simulink model "DroneModel"  (R2023a)
settings: Solver=VariableStepAuto  StartTime=0.0  StopTime=10  RelTol=1e-3
values from neighbouring files (symbols this model uses):
  b = 0.11    [quadraptorModel.m]
  I = diag([Ixx, Iyy, Izz])    [quadraptorModel.m]
  k = 2.165856918e-8    (= 2.165856918e-08)    [quadraptorModel.m]
  L = 0.0475    [quadraptorModel.m]
  m = drone_mass + optitrack_frame_mass    (= 0.067)    [quadraptorModel.m]
  mg = [0; 0; m * g]    [quadraptorModel.m]
  motor_max_rpm = 24000    [quadraptorModel.m]
libraries: slpidlib x2, matrix_library x1
settings Model: Creator=enriq  LastModifiedBy=enriq

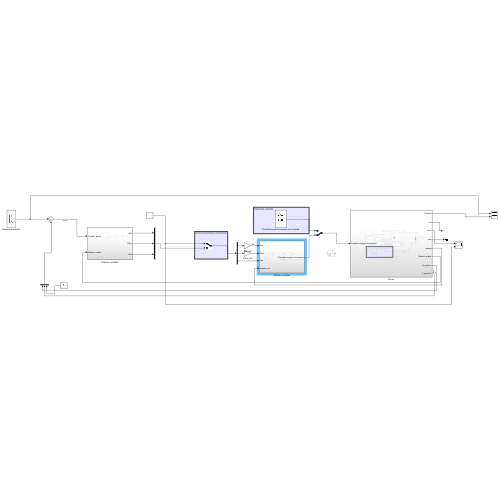
[thumbnail: Simulink's stored preview of the top-level diagram]
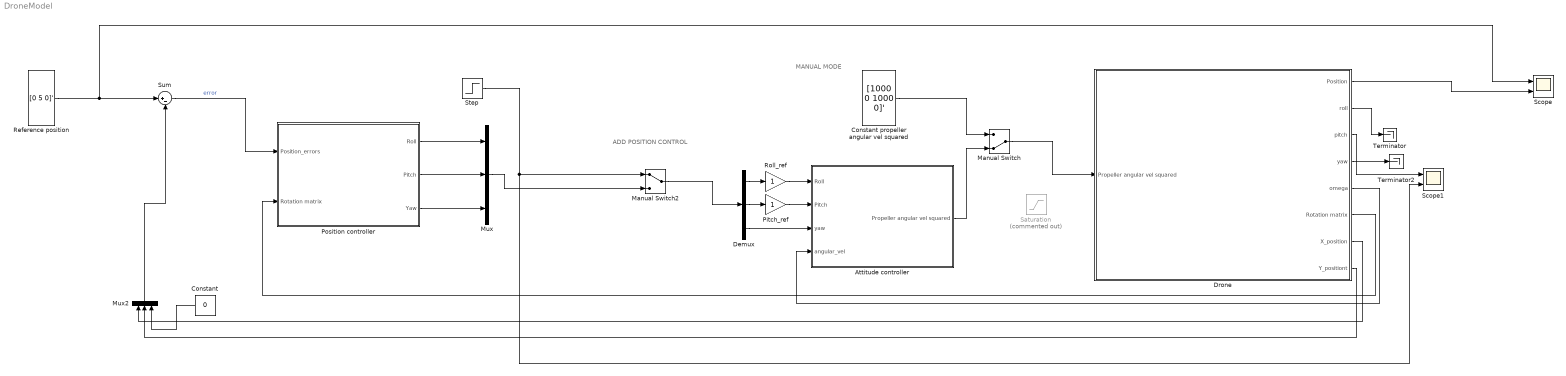
== system DroneModel ==
  note: ADD POSITION CONTROL
  note: MANUAL MODE
  Attitude controller : Subsystem
  Constant : Constant  Value=0
  Constant propeller angular vel squared : Constant  Value=[1000 0 1000 0]'  VectorParams1D=off
  Demux : Demux  Outputs=3
  Drone : Subsystem
  Manual Switch : ManualSwitch  CurrentSetting=0
  Manual Switch2 : ManualSwitch
  Mux : Mux  Inputs=3
  Mux2 : Mux  Inputs=3
  Pitch_ref : Gain
  Position controller : Subsystem
  Reference position : Constant  Value=[0 5 0]'  VectorParams1D=off
  Roll_ref : Gain
  Saturation : Saturate  Commented=on  UpperLimit=motor_max_rpm * (60/(2*pi))
  Scope : Scope  NumInputPorts=2
  Scope1 : Scope  NumInputPorts=2
  Step : Step  Before=[0; 0; 0]  After=[0; 1; 0]  SampleTime=0  VectorParams1D=off
  Sum : Sum  Inputs=|+-
  Terminator : Terminator
  Terminator2 : Terminator
  wires:
  Drone/1(Position) -> Scope/2
  Drone/2(roll) -> Terminator/1
  Drone/4(yaw) -> Terminator2/1
  Reference position/1 -> Scope/1, Sum/1
  Sum/1 -> Position controller/1(Position_errors)  "error"
  Constant propeller angular vel squared/1 -> Manual Switch/1
  Attitude controller/1(Propeller angular vel squared) -> Manual Switch/2
  Drone/5(omega) -> Attitude controller/4(angular_vel)
  Demux/1 -> Roll_ref/1
  Demux/2 -> Pitch_ref/1
  Demux/3 -> Attitude controller/3(yaw)
  Step/1 -> Manual Switch2/1, Scope1/2
  Drone/3(pitch) -> Scope1/1
  Drone/6(Rotation matrix) -> Position controller/2(Rotation matrix)
  Manual Switch2/1 -> Demux/1
  Position controller/1(Roll) -> Mux/1
  Position controller/2(Pitch) -> Mux/2
  Position controller/3(Yaw) -> Mux/3
  Mux/1 -> Manual Switch2/2
  Drone/8(Y_positiont) -> Mux2/2
  Drone/7(X_position) -> Mux2/1
  Constant/1 -> Mux2/3
  Mux2/1 -> Sum/2
  Pitch_ref/1 -> Attitude controller/2(Pitch)
  Roll_ref/1 -> Attitude controller/1(Roll)
  Manual Switch/1 -> Drone/1(Propeller angular vel squared)

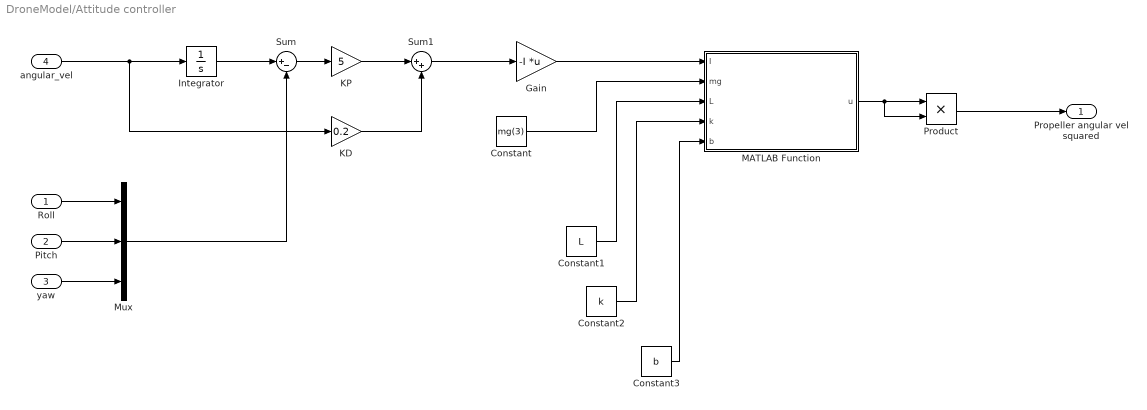
== system DroneModel/Attitude controller ==
  Roll : Inport
  Pitch : Inport  Port=2
  yaw : Inport  Port=3
  angular_vel : Inport  Port=4
  Constant : Constant  Value=mg(3)
  Constant1 : Constant  Value=L
  Constant2 : Constant  Value=k
  Constant3 : Constant  Value=b
  Gain : Gain  Gain=-I  Multiplication=Matrix(K*u)
  Integrator : Integrator
  KD : Gain  Gain=0.2
  KP : Gain  Gain=5
  MATLAB Function : MATLAB Function  TreatAsAtomicUnit=on
  Mux : Mux  Inputs=3
  Product : Product
  Sum : Sum  Inputs=|+-
  Sum1 : Sum  Inputs=|++
  Propeller angular vel squared : Outport
  wires:
  angular_vel/1 -> KD/1, Integrator/1
  Roll/1 -> Mux/1
  Pitch/1 -> Mux/2
  yaw/1 -> Mux/3
  Integrator/1 -> Sum/1
  Mux/1 -> Sum/2
  Sum/1 -> KP/1
  KP/1 -> Sum1/1
  KD/1 -> Sum1/2
  Sum1/1 -> Gain/1
  Gain/1 -> MATLAB Function/1(I)
  Constant1/1 -> MATLAB Function/3(L)
  Constant2/1 -> MATLAB Function/4(k)
  Constant3/1 -> MATLAB Function/5(b)
  MATLAB Function/1(u) -> Product/2, Product/1
  Product/1 -> Propeller angular vel squared/1
  Constant/1 -> MATLAB Function/2(mg)

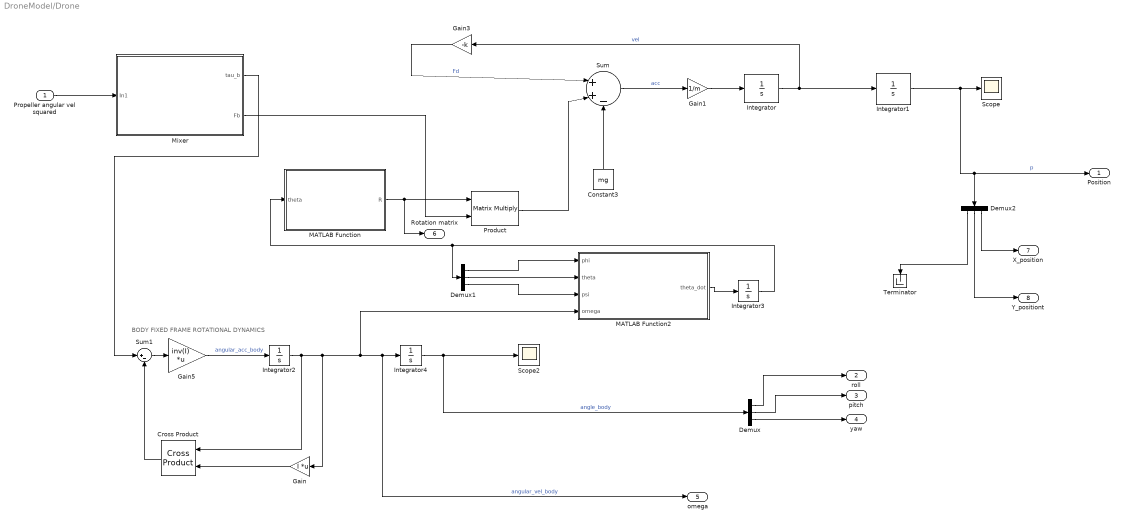
== system DroneModel/Drone ==
  note: BODY FIXED FRAME ROTATIONAL DYNAMICS
  Propeller angular vel squared : Inport
  Constant3 : Constant  Value=mg
  Cross Product : matrix_library/Cross Product
  Demux : Demux  Outputs=3
  Demux1 : Demux  Outputs=3
  Demux2 : Demux  Outputs=3
  Gain : Gain  Gain=I  Multiplication=Matrix(K*u)
  Gain1 : Gain  Gain=1/m
  Gain3 : Gain  Gain=-k
  Gain5 : Gain  Gain=inv(I)  Multiplication=Matrix(K*u)
  Integrator{,1..4} (5 alike) : Integrator
  MATLAB Function : MATLAB Function  TreatAsAtomicUnit=on
  MATLAB Function2 : MATLAB Function  TreatAsAtomicUnit=on
  Mixer : Subsystem
  Product : Product  Multiplication=Matrix(*)
  Scope : Scope
  Scope2 : Scope
  Sum : Sum  Inputs=|++-
  Sum1 : Sum  Inputs=|+-
  Terminator : Terminator
  Position : Outport
  roll : Outport  Port=2
  pitch : Outport  Port=3
  yaw : Outport  Port=4
  omega : Outport  Port=5
  Rotation matrix : Outport  Port=6
  X_position : Outport  Port=7
  Y_positiont : Outport  Port=8
  wires:
  Integrator2/1 -> MATLAB Function2/4(omega), omega/1, Integrator4/1, Gain/1, Cross Product/1  "angular_vel_body"
  Sum1/1 -> Gain5/1
  Mixer/1(tau_b) -> Sum1/1
  Integrator1/1 -> Demux2/1, Position/1, Scope/1  "p"
  Integrator/1 -> Gain3/1, Integrator1/1  "vel"
  Gain/1 -> Cross Product/2
  Integrator3/1 -> Demux1/1, MATLAB Function/1(theta)
  Sum/1 -> Gain1/1  "acc"
  Gain1/1 -> Integrator/1
  Constant3/1 -> Sum/3
  Demux/1 -> roll/1
  Demux/2 -> pitch/1
  Demux/3 -> yaw/1
  Propeller angular vel squared/1 -> Mixer/1(In1)
  MATLAB Function/1(R) -> Rotation matrix/1, Product/1
  Mixer/2(Fb) -> Product/2
  Product/1 -> Sum/2
  Gain3/1 -> Sum/1  "Fd"
  Gain5/1 -> Integrator2/1  "angular_acc_body"
  Cross Product/1 -> Sum1/2
  Integrator4/1 -> Demux/1, Scope2/1  "angle_body"
  MATLAB Function2/1(theta_dot) -> Integrator3/1
  Demux1/1 -> MATLAB Function2/1(phi)
  Demux1/2 -> MATLAB Function2/2(theta)
  Demux1/3 -> MATLAB Function2/3(psi)
  Demux2/3 -> X_position/1
  Demux2/2 -> Y_positiont/1
  Demux2/1 -> Terminator/1

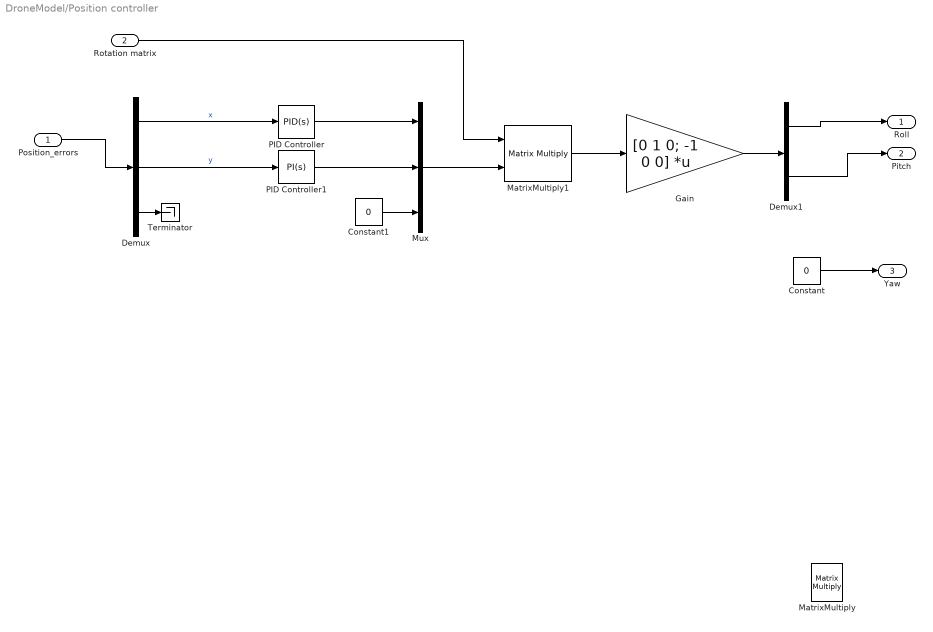
== system DroneModel/Position controller ==
  Position_errors : Inport
  Rotation matrix : Inport  Port=2
  Constant : Constant  Value=0
  Constant1 : Constant  Value=0
  Demux : Demux  Outputs=3
  Demux1 : Demux  Outputs=2
  Gain : Gain  Gain=[0 1 0; -1 0 0]  Multiplication=Matrix(K*u)
  MatrixMultiply : Product  Multiplication=Matrix(*)
  MatrixMultiply1 : Product  Multiplication=Matrix(*)
  Mux : Mux  Inputs=3
  PID Controller : slpidlib/PID Controller  Controller=PID  Form=Parallel  TimeDomain=Continuous-time  UseExternalTs=off  SampleTime=-1  IntegratorMethod=Forward Euler  FilterMethod=Forward Euler  ControllerParametersSource=internal  P=1  I=1  UseKiTs=off  D=0  N=100  UseFilter=on  TunerSelectOption=Transfer Function Based (PID Tuner App)  InitialConditionSource=internal  InitialConditionForIntegrator=0  InitialConditionForFilter=0  DifferentiatorICPrevScaledInput=0  ExternalReset=none  TrackingMode=off  Kt=1  LimitOutput=off  SatLimitsSource=internal  UpperSaturationLimit=inf  LowerSaturationLimit=-inf  LinearizeAsGain=on  AntiWindupMode=none  Kb=1  LimitIntegrator=off  UpperIntegratorSaturationLimit=inf  LowerIntegratorSaturationLimit=-inf  POutMin=[]  POutMax=[]  IOutMin=[]  IOutMax=[]  DOutMin=[]  DOutMax=[]  NOutMin=[]  NOutMax=[]  SumOutMin=[]  SumOutMax=[]  SaturationOutMin=[]  SaturationOutMax=[]  PParamMin=[]  PParamMax=[]  IParamMin=[]  IParamMax=[]  DParamMin=[]  DParamMax=[]  NParamMin=[]  NParamMax=[]  KbParamMin=[]  KbParamMax=[]  KtParamMin=[]  KtParamMax=[]  KbOutMin=[]  KbOutMax=[]  KtOutMin=[]  KtOutMax=[]  IntegratorOutMin=[]  IntegratorOutMax=[]  FilterOutMin=[]  FilterOutMax=[]  SumI1OutMin=[]  SumI1OutMax=[]  SumI2OutMin=[]  SumI2OutMax=[]  SumI3OutMin=[]  SumI3OutMax=[]  SumI4OutMin=[]  SumI4OutMax=[]  SumDOutMin=[]  SumDOutMax=[]  DifferentiatorOutMin=[]  DifferentiatorOutMax=[]  FilterDiffOutCoefMin=[]  FilterDiffOutCoefMax=[]  ReciprocalOutMin=[]  ReciprocalOutMax=[]  SumDenOutMin=[]  SumDenOutMax=[]  SumNumOutMin=[]  SumNumOutMax=[]  DivideOutMin=[]  DivideOutMax=[]  UdiffTsProdOutMin=[]  UdiffTsProdOutMax=[]  NTsProdOutMin=[]  NTsProdOutMax=[]  UintegralTsProdOutMin=[]  UintegralTsProdOutMax=[]  UngainTsProdOutMin=[]  UngainTsProdOutMax=[]  ClampingZeroOutDataTypeStr=Inherit: Inherit via back propagation  ClampingZeroOutMin=[]  ClampingZeroOutMax=[]  FilterDenConstantOutDataTypeStr=Inherit: Inherit via back propagation  FilterDenConstantOutMin=[]  FilterDenConstantOutMax=[]  PCopyOutDataTypeStr=Inherit: Inherit via back propagation  PCopyOutMin=[]  PCopyOutMax=[]  NCopyOutDataTypeStr=Inherit: Inherit via back propagation  NCopyOutMin=[]  NCopyOutMax=[]  IntegratorContinuousStateAttributes=''  IntegratorStateMustResolveToSignalObject=off  IntegratorRTWStateStorageClass=Auto  FilterContinuousStateAttributes=''  FilterStateMustResolveToSignalObject=off  FilterRTWStateStorageClass=Auto  ParallelPVariant=InternalParameters  IdealPVariant=Disabled  IVariant=InternalParameters  DVariant=InternalParameters  IntegratorVariant=Continuous  SatVariant=Disabled  AWVariant=Passthrough  PCopyVariant=Disabled  TRVariant=Disabled  FdbkBlocksVariant=Forward  IdealPFdbkVariant=Disabled  SatFdbkVariant=Disabled  DerivativeFilterVariant=ContFilter  NVariant=InternalParameters  NCopyVariant=Disabled  FilterICVariant=InternalICsFilter  IntegratorICVariant=InternalICs  ExternalResetVariant=Disabled  TRSumVariant=Passthrough  SumFdbkVariant=Disabled  SumVariant=Sum_PID  TsampFilterVariant=InternalTs  TsampNgainVariant=Passthrough  TsampIntegralVariant=Disabled_SignalSpec  ExternalSaturationOutDataTypeStr=Inherit: Same as second input
  PID Controller1 : slpidlib/PID Controller  Controller=PI  Form=Parallel  TimeDomain=Continuous-time  UseExternalTs=off  SampleTime=-1  IntegratorMethod=Forward Euler  FilterMethod=Forward Euler  ControllerParametersSource=internal  P=4.65  I=1  UseKiTs=off  D=0  N=100  UseFilter=on  TunerSelectOption=Transfer Function Based (PID Tuner App)  InitialConditionSource=internal  InitialConditionForIntegrator=0  InitialConditionForFilter=0  DifferentiatorICPrevScaledInput=0  ExternalReset=none  TrackingMode=off  Kt=1  LimitOutput=off  SatLimitsSource=internal  UpperSaturationLimit=inf  LowerSaturationLimit=-inf  LinearizeAsGain=on  AntiWindupMode=none  Kb=1  LimitIntegrator=off  UpperIntegratorSaturationLimit=inf  LowerIntegratorSaturationLimit=-inf  POutMin=[]  POutMax=[]  IOutMin=[]  IOutMax=[]  DOutMin=[]  DOutMax=[]  NOutMin=[]  NOutMax=[]  SumOutMin=[]  SumOutMax=[]  SaturationOutMin=[]  SaturationOutMax=[]  PParamMin=[]  PParamMax=[]  IParamMin=[]  IParamMax=[]  DParamMin=[]  DParamMax=[]  NParamMin=[]  NParamMax=[]  KbParamMin=[]  KbParamMax=[]  KtParamMin=[]  KtParamMax=[]  KbOutMin=[]  KbOutMax=[]  KtOutMin=[]  KtOutMax=[]  IntegratorOutMin=[]  IntegratorOutMax=[]  FilterOutMin=[]  FilterOutMax=[]  SumI1OutMin=[]  SumI1OutMax=[]  SumI2OutMin=[]  SumI2OutMax=[]  SumI3OutMin=[]  SumI3OutMax=[]  SumI4OutMin=[]  SumI4OutMax=[]  SumDOutMin=[]  SumDOutMax=[]  DifferentiatorOutMin=[]  DifferentiatorOutMax=[]  FilterDiffOutCoefMin=[]  FilterDiffOutCoefMax=[]  ReciprocalOutMin=[]  ReciprocalOutMax=[]  SumDenOutMin=[]  SumDenOutMax=[]  SumNumOutMin=[]  SumNumOutMax=[]  DivideOutMin=[]  DivideOutMax=[]  UdiffTsProdOutMin=[]  UdiffTsProdOutMax=[]  NTsProdOutMin=[]  NTsProdOutMax=[]  UintegralTsProdOutMin=[]  UintegralTsProdOutMax=[]  UngainTsProdOutMin=[]  UngainTsProdOutMax=[]  ClampingZeroOutDataTypeStr=Inherit: Inherit via back propagation  ClampingZeroOutMin=[]  ClampingZeroOutMax=[]  FilterDenConstantOutDataTypeStr=Inherit: Inherit via back propagation  FilterDenConstantOutMin=[]  FilterDenConstantOutMax=[]  PCopyOutDataTypeStr=Inherit: Inherit via back propagation  PCopyOutMin=[]  PCopyOutMax=[]  NCopyOutDataTypeStr=Inherit: Inherit via back propagation  NCopyOutMin=[]  NCopyOutMax=[]  IntegratorContinuousStateAttributes=''  IntegratorStateMustResolveToSignalObject=off  IntegratorRTWStateStorageClass=Auto  FilterContinuousStateAttributes=''  FilterStateMustResolveToSignalObject=off  FilterRTWStateStorageClass=Auto  ParallelPVariant=InternalParameters  IdealPVariant=Disabled  IVariant=InternalParameters  DVariant=Disabled  IntegratorVariant=Continuous  SatVariant=Disabled  AWVariant=Passthrough  PCopyVariant=Disabled  TRVariant=Disabled  FdbkBlocksVariant=Forward  IdealPFdbkVariant=Disabled  SatFdbkVariant=Disabled  DerivativeFilterVariant=Disabled  NVariant=Disabled  NCopyVariant=Disabled_SignalSpec  FilterICVariant=Disabled  IntegratorICVariant=InternalICs  ExternalResetVariant=Disabled  TRSumVariant=Passthrough  SumFdbkVariant=Disabled  SumVariant=Sum_PI  TsampFilterVariant=InternalTs  TsampNgainVariant=Passthrough  TsampIntegralVariant=Disabled_SignalSpec  ExternalSaturationOutDataTypeStr=Inherit: Same as second input
  Terminator : Terminator
  Roll : Outport
  Pitch : Outport  Port=2
  Yaw : Outport  Port=3
  wires:
  Constant/1 -> Yaw/1
  Position_errors/1 -> Demux/1
  Demux/1 -> PID Controller/1  "x"
  Demux/2 -> PID Controller1/1  "y"
  Demux/3 -> Terminator/1
  PID Controller/1 -> Mux/1
  PID Controller1/1 -> Mux/2
  Constant1/1 -> Mux/3
  Rotation matrix/1 -> MatrixMultiply1/1
  Mux/1 -> MatrixMultiply1/2
  MatrixMultiply1/1 -> Gain/1
  Gain/1 -> Demux1/1
  Demux1/1 -> Roll/1
  Demux1/2 -> Pitch/1

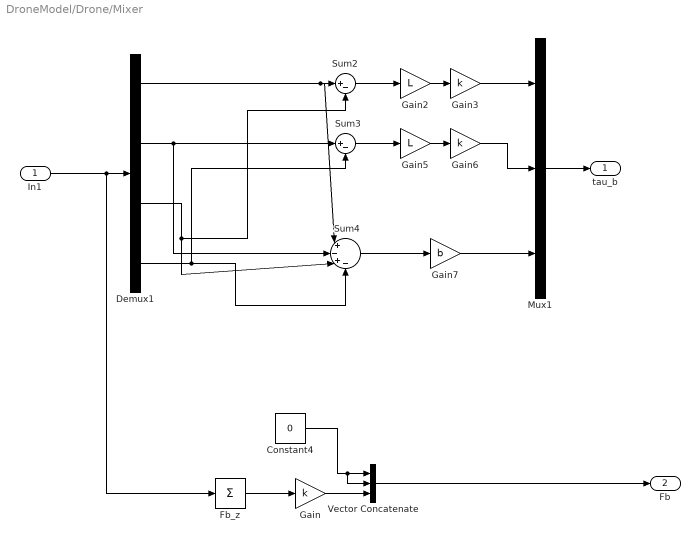
== system DroneModel/Drone/Mixer ==
  In1 : Inport
  Constant4 : Constant  Value=0
  Demux1 : Demux
  Fb_z : Sum  Inputs=+
  Gain : Gain  Gain=k
  Gain2 : Gain  Gain=L
  Gain3 : Gain  Gain=k
  Gain5 : Gain  Gain=L
  Gain6 : Gain  Gain=k
  Gain7 : Gain  Gain=b
  Mux1 : Mux  Inputs=3
  Sum2 : Sum  Inputs=|+-
  Sum3 : Sum  Inputs=|+-
  Sum4 : Sum  Inputs=|+-+-
  Vector Concatenate : Concatenate  NumInputs=3
  tau_b : Outport
  Fb : Outport  Port=2
  wires:
  Sum4/1 -> Gain7/1
  Demux1/2 -> Sum3/1, Sum4/2
  Sum2/1 -> Gain2/1
  Mux1/1 -> tau_b/1
  Demux1/3 -> Sum4/3, Sum2/2
  Demux1/1 -> Sum2/1, Sum4/1
  Demux1/4 -> Sum4/4, Sum3/2
  Sum3/1 -> Gain5/1
  Gain2/1 -> Gain3/1
  Gain5/1 -> Gain6/1
  Gain3/1 -> Mux1/1
  Gain7/1 -> Mux1/3
  Gain6/1 -> Mux1/2
  Constant4/1 -> Vector Concatenate/2, Vector Concatenate/1
  Fb_z/1 -> Gain/1
  In1/1 -> Fb_z/1, Demux1/1
  Vector Concatenate/1 -> Fb/1
  Gain/1 -> Vector Concatenate/3

== matlab function DroneModel/Attitude controller/MATLAB Function ==
  data: I input; u output; mg input; L input; k input; b input
function u = computeControlAction(I, mg, L, k, b)

I = [I; mg/k];

A = [L*k,  0,  -L*k,   0;
     0,   L*k,  0,   -L*k;
     b,   -b,   b,     -b;
     1,    1,   1,      1];

u = A\I;

== matlab function DroneModel/Drone/MATLAB Function ==
  data: theta input; R output
function R = computeRotationMatrix(theta)

Rx = [1     0               0;
      0 cos(theta(1)) -sin(theta(1));
      0 sin(theta(1))  cos(theta(1))];

Ry = [cos(theta(2))     0         sin(theta(2));
      0                 1               0;
      -sin(theta(2))    0         cos(theta(2))];

Rz = [cos(theta(3)) -sin(theta(3))    0;
      sin(theta(3))  cos(theta(3))    0;
          0               0           1];


R = Rx * Ry * Rz;

== matlab function DroneModel/Drone/MATLAB Function2 ==
  data: phi input; theta input; psi input; theta_dot output; omega input
function theta_dot = getAngularVelocityFixedFrame(phi, theta, psi, omega)



A = [1, 0, -sin(theta);
     0, cos(phi), cos(theta) * sin(phi);
     0, -sin(phi), cos(theta) * cos(phi)];

theta_dot = inv(A)* omega;
